simulink library "BrickPi"  (R2018b)
settings: Solver=VariableStepAuto  StartTime=0.0  StopTime=10.0  RelTol=1e-3
libraries: raspberrypilib x50, hdlsllib x27, xpcutilitieslib x18, $bdroot x1
(part 3 of 4)

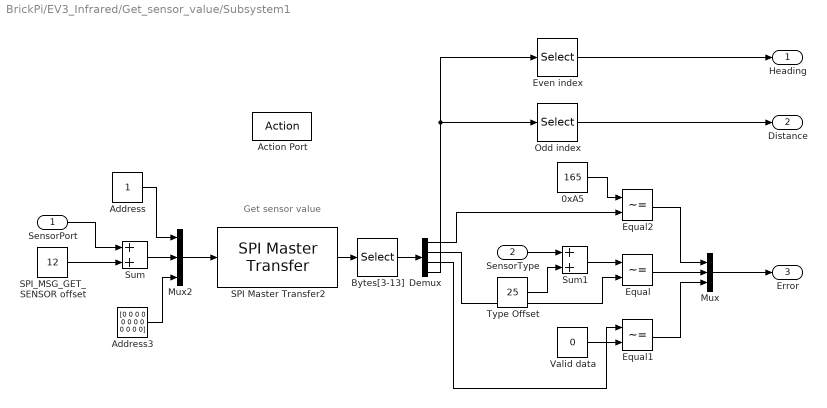
== system BrickPi/EV3_Infrared/Get_sensor_value/Subsystem1 ==
  note: Get sensor value
  SensorPort : Inport
  SensorType : Inport  Port=2  OutDataTypeStr=uint8
  Action Port : ActionPort  ActionType=case
  0xA5 : Constant  Value=165
  "Address " : Constant  OutDataTypeStr=uint8
  Address3 : Constant  Value=[0 0 0 0 0 0 0 0 0 0 0 0]  OutDataTypeStr=uint8
  Bytes[3-13] : Selector  IndexMode=Zero-based  InputPortWidth=14  IndexOptions=Index vector (dialog)  Indices=[3 4 5 6 7 8 9 10 11 12 13]  OutputSizes=1
  Demux : Demux
  Equal : RelationalOperator  Operator=~=  OutDataTypeStr=boolean  RndMeth=Simplest
  Equal1 : RelationalOperator  Operator=~=  OutDataTypeStr=boolean  RndMeth=Simplest
  Equal2 : RelationalOperator  Operator=~=  OutDataTypeStr=boolean  RndMeth=Simplest
  Even index : Selector  IndexMode=Zero-based  InputPortWidth=8  IndexOptions=Index vector (dialog)  Indices=[0 2 4 6]  OutputSizes=1
  Mux : Mux  Inputs=3
  Mux2 : Mux  Inputs=3
  Odd index : Selector  IndexMode=Zero-based  InputPortWidth=8  IndexOptions=Index vector (dialog)  Indices=[1 3 5 7]  OutputSizes=1
  SPI Master Transfer2 : raspberrypilib/SPI Master Transfer  Priority=6  BoardProperty=Pi 3 Model B  SPIModule=uint32(0)  Mode=Master  BusSpeed=1000000  Pin=SPI0_CE1  FirstBitToTransfer=Most significant bit (MSB)  ClockMode=0  BlockFunction=Transfer  RegisterAddress=0  OutputDataType=int8  OutputDataLength=1
      settings: SourceProductName=Simulink Support Package for Raspberry Pi Hardware  SourceProductBaseCode=RASPPI
  SPI_MSG_GET_ SENSOR offset : Constant  Value=12  OutMin=[1]  OutMax=[28]  OutDataTypeStr=uint8
  Sum : Sum  OutDataTypeStr=uint8
  Sum1 : Sum  OutDataTypeStr=uint8
  Type Offset : Constant  Value=25  OutDataTypeStr=uint8
  Valid data : Constant  Value=0  OutDataTypeStr=uint8
  Heading : Outport
  Distance : Outport  Port=2
  Error : Outport  Port=3
  wires:
  Equal2/1 -> Mux/1
  Demux/1 -> Equal2/2
  SPI_MSG_GET_ SENSOR offset/1 -> Sum/2
  Demux/3 -> Equal1/1
  Equal/1 -> Mux/2
  Demux/2 -> Equal/2
  Equal1/1 -> Mux/3
  "Address "/1 -> Mux2/1
  Valid data/1 -> Equal1/2
  Mux/1 -> Error/1
  Mux2/1 -> SPI Master Transfer2/1
  SPI Master Transfer2/1 -> Bytes[3-13]/1
  Bytes[3-13]/1 -> Demux/1
  Address3/1 -> Mux2/3
  SensorPort/1 -> Sum/1
  Sum/1 -> Mux2/2
  0xA5/1 -> Equal2/1
  Demux/4 -> Odd index/1, Even index/1
  Odd index/1 -> Distance/1
  Even index/1 -> Heading/1
  SensorType/1 -> Sum1/1
  Type Offset/1 -> Sum1/2
  Sum1/1 -> Equal/1

== system BrickPi/EV3_Infrared/Get_sensor_value/Subsystem2 ==
  note: Get sensor value
  SensorPort : Inport
  SensorType : Inport  Port=2  OutDataTypeStr=uint8
  Action Port : ActionPort  ActionType=case
  0xA5 : Constant  Value=165
  "Address " : Constant  OutDataTypeStr=uint8
  Address3 : Constant  Value=[0 0 0 0 0 0 0 0]  OutDataTypeStr=uint8
  Bytes[3-9] : Selector  IndexMode=Zero-based  InputPortWidth=10  IndexOptions=Index vector (dialog)  Indices=[3 4 5 6 7 8 9]  OutputSizes=1
  Demux : Demux
  Equal : RelationalOperator  Operator=~=  OutDataTypeStr=boolean  RndMeth=Simplest
  Equal1 : RelationalOperator  Operator=~=  OutDataTypeStr=boolean  RndMeth=Simplest
  Equal2 : RelationalOperator  Operator=~=  OutDataTypeStr=boolean  RndMeth=Simplest
  Mux : Mux  Inputs=3
  Mux2 : Mux  Inputs=3
  SPI Master Transfer2 : raspberrypilib/SPI Master Transfer  Priority=6  BoardProperty=Pi 3 Model B  SPIModule=uint32(0)  Mode=Master  BusSpeed=1000000  Pin=SPI0_CE1  FirstBitToTransfer=Most significant bit (MSB)  ClockMode=0  BlockFunction=Transfer  RegisterAddress=0  OutputDataType=int8  OutputDataLength=1
      settings: SourceProductName=Simulink Support Package for Raspberry Pi Hardware  SourceProductBaseCode=RASPPI
  SPI_MSG_GET_ SENSOR offset : Constant  Value=12  OutMin=[1]  OutMax=[28]  OutDataTypeStr=uint8
  Sum : Sum  OutDataTypeStr=uint8
  Sum1 : Sum  OutDataTypeStr=uint8
  Type Offset : Constant  Value=25  OutDataTypeStr=uint8
  Valid data : Constant  Value=0  OutDataTypeStr=uint8
  Remote : Outport
  Error : Outport  Port=2
  wires:
  Sum1/1 -> Equal/1
  Type Offset/1 -> Sum1/2
  SensorType/1 -> Sum1/1
  Demux/4 -> Remote/1
  0xA5/1 -> Equal2/1
  Sum/1 -> Mux2/2
  SensorPort/1 -> Sum/1
  Address3/1 -> Mux2/3
  Bytes[3-9]/1 -> Demux/1
  SPI Master Transfer2/1 -> Bytes[3-9]/1
  Mux2/1 -> SPI Master Transfer2/1
  Mux/1 -> Error/1
  Valid data/1 -> Equal1/2
  "Address "/1 -> Mux2/1
  Equal1/1 -> Mux/3
  Demux/2 -> Equal/2
  Equal/1 -> Mux/2
  Demux/3 -> Equal1/1
  SPI_MSG_GET_ SENSOR offset/1 -> Sum/2
  Demux/1 -> Equal2/2
  Equal2/1 -> Mux/1

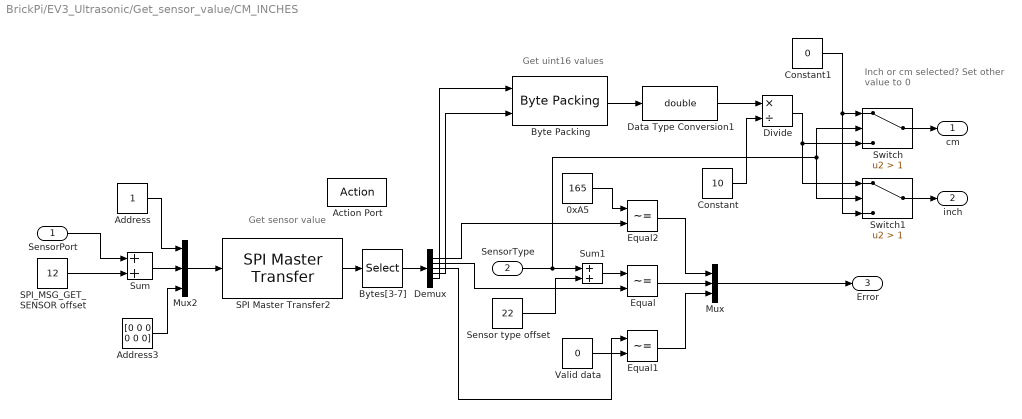
== system BrickPi/EV3_Ultrasonic/Get_sensor_value/CM_INCHES ==
  note: Inch or cm selected?
      | Set other value to 0
  note: Get uint16 values
  note: Get sensor value
  SensorPort : Inport
  SensorType : Inport  Port=2  OutDataTypeStr=uint8
  Action Port : ActionPort  ActionType=case
  0xA5 : Constant  Value=165
  "Address " : Constant  OutDataTypeStr=uint8
  Address3 : Constant  Value=[0 0 0 0 0 0]  OutDataTypeStr=uint8
  "Byte Packing " : xpcutilitieslib/Byte Packing   MaskPackedDataType=uint16  MaskUnpackedDataTypes={'uint8','uint8'}  MaskAlignment=1
  Bytes[3-7] : Selector  IndexMode=Zero-based  InputPortWidth=8  IndexOptions=Index vector (dialog)  Indices=[3 4 5 6 7]  OutputSizes=1
  Constant : Constant  Value=10
  Constant1 : Constant  Value=0
  Data Type Conversion1 : DataTypeConversion  OutDataTypeStr=double
  Demux : Demux  Outputs=5
  Divide : Product  Inputs=*/
  Equal : RelationalOperator  Operator=~=  OutDataTypeStr=boolean  RndMeth=Simplest
  Equal1 : RelationalOperator  Operator=~=  OutDataTypeStr=boolean  RndMeth=Simplest
  Equal2 : RelationalOperator  Operator=~=  OutDataTypeStr=boolean  RndMeth=Simplest
  Mux : Mux  Inputs=3
  Mux2 : Mux  Inputs=3
  SPI Master Transfer2 : raspberrypilib/SPI Master Transfer  Priority=6  BoardProperty=Pi 3 Model B  SPIModule=uint32(0)  Mode=Master  BusSpeed=1000000  Pin=SPI0_CE1  FirstBitToTransfer=Most significant bit (MSB)  ClockMode=0  BlockFunction=Transfer  RegisterAddress=0  OutputDataType=int8  OutputDataLength=1
      settings: SourceProductName=Simulink Support Package for Raspberry Pi Hardware  SourceProductBaseCode=RASPPI
  SPI_MSG_GET_ SENSOR offset : Constant  Value=12  OutMin=[1]  OutMax=[28]  OutDataTypeStr=uint8
  Sensor type offset : Constant  Value=22  OutDataTypeStr=uint8
  Sum : Sum  OutDataTypeStr=uint8
  Sum1 : Sum
  Switch : Switch  Criteria=u2 > Threshold  Threshold=1
  Switch1 : Switch  Criteria=u2 > Threshold  Threshold=1
  Valid data : Constant  Value=0  OutDataTypeStr=uint8
  cm : Outport
  inch : Outport  Port=2
  Error : Outport  Port=3
  wires:
  0xA5/1 -> Equal2/1
  Equal1/1 -> Mux/3
  Equal2/1 -> Mux/1
  SPI Master Transfer2/1 -> Bytes[3-7]/1
  SensorType/1 -> Switch/2, Switch1/2, Sum1/1
  "Address "/1 -> Mux2/1
  Sum/1 -> Mux2/2
  Sensor type offset/1 -> Sum1/2
  Address3/1 -> Mux2/3
  Demux/2 -> Equal/2
  Mux2/1 -> SPI Master Transfer2/1
  Valid data/1 -> Equal1/2
  Demux/3 -> Equal1/1
  Sum1/1 -> Equal/1
  Mux/1 -> Error/1
  SPI_MSG_GET_ SENSOR offset/1 -> Sum/2
  Demux/1 -> Equal2/2
  Bytes[3-7]/1 -> Demux/1
  SensorPort/1 -> Sum/1
  Equal/1 -> Mux/2
  "Byte Packing "/1 -> Data Type Conversion1/1
  Data Type Conversion1/1 -> Divide/1
  Constant/1 -> Divide/2
  Switch/1 -> cm/1
  Switch1/1 -> inch/1
  Divide/1 -> Switch/3, Switch1/1
  Constant1/1 -> Switch/1, Switch1/3
  Demux/4 -> "Byte Packing "/2
  Demux/5 -> "Byte Packing "/1

== system BrickPi/EV3_Ultrasonic/Get_sensor_value/LISTEN ==
  note: Get sensor value
  SensorPort : Inport
  Action Port : ActionPort  ActionType=case
  0xA5 : Constant  Value=165
  "Address " : Constant  OutDataTypeStr=uint8
  Address3 : Constant  Value=[0 0 0 0 0]  OutDataTypeStr=uint8
  Bytes[3-6] : Selector  IndexMode=Zero-based  InputPortWidth=7  IndexOptions=Index vector (dialog)  Indices=[3 4 5 6]  OutputSizes=1
  Cast To Boolean : DataTypeConversion  OutDataTypeStr=boolean
  Demux : Demux
  Mux : Mux  Inputs=3
  Mux2 : Mux  Inputs=3
  NAND : Logic  Operator=NAND  IconShape=distinctive  AllPortsSameDT=off  OutDataTypeStr=boolean
  NAND1 : Logic  Operator=NAND  IconShape=distinctive  AllPortsSameDT=off  OutDataTypeStr=boolean
  OR1 : Logic  Operator=OR  IconShape=distinctive  AllPortsSameDT=off  OutDataTypeStr=boolean
  SPI Master Transfer2 : raspberrypilib/SPI Master Transfer  Priority=6  BoardProperty=Pi 3 Model B  SPIModule=uint32(0)  Mode=Master  BusSpeed=1000000  Pin=SPI0_CE1  FirstBitToTransfer=Most significant bit (MSB)  ClockMode=0  BlockFunction=Transfer  RegisterAddress=0  OutputDataType=int8  OutputDataLength=1
      settings: SourceProductName=Simulink Support Package for Raspberry Pi Hardware  SourceProductBaseCode=RASPPI
  SPI_MSG_GET_ SENSOR offset : Constant  Value=12  OutMin=[1]  OutMax=[28]  OutDataTypeStr=uint8
  Sum : Sum  OutDataTypeStr=uint8
  ULTRASONIC_LISTEN : Constant  Value=25  OutMin=[1]  OutMax=[28]  OutDataTypeStr=uint8
  Valid data : Constant  Value=0  OutDataTypeStr=uint8
  presence : Outport
  Error : Outport  Port=2
  wires:
  ULTRASONIC_LISTEN/1 -> NAND1/1
  NAND/1 -> Mux/1
  SPI Master Transfer2/1 -> Bytes[3-6]/1
  Valid data/1 -> OR1/2
  Sum/1 -> Mux2/2
  0xA5/1 -> NAND/1
  Demux/3 -> OR1/1
  Mux2/1 -> SPI Master Transfer2/1
  Address3/1 -> Mux2/3
  NAND1/1 -> Mux/2
  Demux/2 -> NAND1/2
  "Address "/1 -> Mux2/1
  Demux/4 -> Cast To Boolean/1
  Demux/1 -> NAND/2
  SensorPort/1 -> Sum/1
  SPI_MSG_GET_ SENSOR offset/1 -> Sum/2
  Mux/1 -> Error/1
  OR1/1 -> Mux/3
  Bytes[3-6]/1 -> Demux/1
  Cast To Boolean/1 -> presence/1

== system BrickPi/Motor_Encoder/Get Encoder Value/Switch Case Action Subsystem ==
  note: Change from zero to nonzero?
  note: Change in input signal?
  ExtSignal : Inport
  MotorPort : Inport  Port=2
  Action Port : ActionPort  ActionType=case
  AND : Logic  IconShape=distinctive  AllPortsSameDT=off  OutDataTypeStr=boolean
  Constant : Constant  Value=0
  Equal : RelationalOperator  Operator=~=  OutDataTypeStr=boolean  RndMeth=Simplest
  Equal1 : RelationalOperator  Operator=~=  OutDataTypeStr=boolean  RndMeth=Simplest
  Memory : Memory
  Subsystem : Subsystem
  wires:
  Equal/1 -> AND/1
  Equal1/1 -> AND/2
  Memory/1 -> Equal/1
  Constant/1 -> Equal1/2
  ExtSignal/1 -> Equal1/1, Equal/2, Memory/1
  AND/1 -> Subsystem/Enable
  MotorPort/1 -> Subsystem/1(MotorPort)

== system BrickPi/Motor_Encoder/Reset Encoder once/Encoder ==
  note: Get motor encoder
  MotorPort : Inport
  0xA5 : Constant  Value=165
  "Address " : Constant  OutDataTypeStr=uint8
  Address3 : Constant  Value=[0 0 0 0 0 0 0 0]  OutDataTypeStr=uint8
  "Byte Packing " : xpcutilitieslib/Byte Packing   MaskPackedDataType=int32  MaskUnpackedDataTypes={'uint8', 'uint8', 'uint8', 'uint8'}  MaskAlignment=1
  Bytes[3-7] : Selector  IndexMode=Zero-based  InputPortWidth=10  IndexOptions=Index vector (dialog)  Indices=[3 4 5 6 7]  OutputSizes=1
  Demux : Demux  Outputs=5
  Mux2 : Mux  Inputs=3
  NAND : Logic  Operator=NAND  IconShape=distinctive  AllPortsSameDT=off  OutDataTypeStr=boolean
  SPI Master Transfer2 : raspberrypilib/SPI Master Transfer  Priority=6  BoardProperty=Pi 3 Model B  SPIModule=uint32(0)  Mode=Master  BusSpeed=1000000  Pin=SPI0_CE1  FirstBitToTransfer=Most significant bit (MSB)  ClockMode=0  BlockFunction=Transfer  RegisterAddress=0  OutputDataType=int8  OutputDataLength=1
      settings: SourceProductName=Simulink Support Package for Raspberry Pi Hardware  SourceProductBaseCode=RASPPI
  SPI_MSG_GET_ MOTOR_ENCODER offset : Constant  Value=29  OutDataTypeStr=uint8
  Sum : Sum  OutDataTypeStr=uint8
  Value : Outport
  Error : Outport  Port=2
  wires:
  Address3/1 -> Mux2/3
  NAND/1 -> Error/1
  Sum/1 -> Mux2/2
  Mux2/1 -> SPI Master Transfer2/1
  MotorPort/1 -> Sum/1
  Demux/5 -> "Byte Packing "/1
  "Address "/1 -> Mux2/1
  Demux/4 -> "Byte Packing "/2
  Demux/3 -> "Byte Packing "/3
  Demux/1 -> NAND/2
  0xA5/1 -> NAND/1
  Demux/2 -> "Byte Packing "/4
  "Byte Packing "/1 -> Value/1
  Bytes[3-7]/1 -> Demux/1
  SPI Master Transfer2/1 -> Bytes[3-7]/1
  SPI_MSG_GET_ MOTOR_ENCODER offset/1 -> Sum/2

== system BrickPi/Motor_Encoder/Reset Encoder once/Motor_Offset ==
  note: Set offset value
  Offset : Inport  OutDataTypeStr=int32
  MotorPort : Inport  Port=2  OutDataTypeStr=uint8
  "Address " : Constant  OutDataTypeStr=uint8
  Bit Shift : hdlsllib/Logic and Bit Operations/Bit Shift  mode=Shift Right Logical  N=24
      settings: SourceProductName=HDL Coder  SourceProductBaseCode=HD
  Bit Shift1 : hdlsllib/Logic and Bit Operations/Bit Shift  mode=Shift Right Logical  N=16
      settings: SourceProductName=HDL Coder  SourceProductBaseCode=HD
  Bit Shift2 : hdlsllib/Logic and Bit Operations/Bit Shift  mode=Shift Right Logical  N=8
      settings: SourceProductName=HDL Coder  SourceProductBaseCode=HD
  Constant2 : Constant  OutDataTypeStr=uint8
  Constant3 : Constant  OutDataTypeStr=uint8
  Data Type Conversion{,1..3} (4 alike) : DataTypeConversion  OutDataTypeStr=uint8
  Mux2 : Mux  Inputs=7
  SPI Master Transfer2 : raspberrypilib/SPI Master Transfer  Priority=6  BoardProperty=Pi 3 Model B  SPIModule=uint32(0)  Mode=Master  BusSpeed=1000000  Pin=SPI0_CE1  FirstBitToTransfer=Most significant bit (MSB)  ClockMode=0  BlockFunction=Transfer  RegisterAddress=0  OutputDataType=int8  OutputDataLength=1
      settings: SourceProductName=Simulink Support Package for Raspberry Pi Hardware  SourceProductBaseCode=RASPPI
  SPI_MSG_ OFFSET_ENCODER : Constant  Value=29  OutMin=[1]  OutDataTypeStr=uint8
  Shift Arithmetic : ArithShift  BitShiftNumberSource=Input port  BitShiftNumber=8  BitShiftDirection=Left
      settings: InputPortMap=u0,p1
  Subtract : Sum  Inputs=+-
  Terminator : Terminator
  wires:
  Data Type Conversion/1 -> Mux2/4
  Data Type Conversion2/1 -> Mux2/6
  Offset/1 -> Bit Shift1/1, Bit Shift2/1, Data Type Conversion3/1, Bit Shift/1
  Constant2/1 -> Shift Arithmetic/1
  Bit Shift2/1 -> Data Type Conversion2/1
  Constant3/1 -> Subtract/2
  Bit Shift/1 -> Data Type Conversion/1
  Mux2/1 -> SPI Master Transfer2/1
  SPI Master Transfer2/1 -> Terminator/1
  Data Type Conversion3/1 -> Mux2/7
  Subtract/1 -> Shift Arithmetic/2
  MotorPort/1 -> Subtract/1
  Bit Shift1/1 -> Data Type Conversion1/1
  Data Type Conversion1/1 -> Mux2/5
  SPI_MSG_ OFFSET_ENCODER/1 -> Mux2/2
  "Address "/1 -> Mux2/1
  Shift Arithmetic/1 -> Mux2/3

== system BrickPi/Motor_Power/Subsystem/Set_DPS ==
  note: Get sensor value
  DPS : Inport  OutDataTypeStr=int16
  Action Port : ActionPort  ActionType=case
  "Address " : Constant  OutDataTypeStr=uint8
  Bit Shift : hdlsllib/Logic and Bit Operations/Bit Shift  mode=Shift Right Logical  N=8
      settings: SourceProductName=HDL Coder  SourceProductBaseCode=HD
  Constant2 : Constant  OutDataTypeStr=uint8
  Constant3 : Constant  OutDataTypeStr=uint8
  Data Type Conversion : DataTypeConversion  OutDataTypeStr=uint8
  Data Type Conversion1 : DataTypeConversion  OutDataTypeStr=uint8
  MotorPort : Constant  Value=MotorPort  OutDataTypeStr=uint8
  Mux2 : Mux  Inputs=5
  SPI Master Transfer2 : raspberrypilib/SPI Master Transfer  Priority=6  BoardProperty=Pi 3 Model B  SPIModule=uint32(0)  Mode=Master  BusSpeed=1000000  Pin=SPI0_CE1  FirstBitToTransfer=Most significant bit (MSB)  ClockMode=0  BlockFunction=Transfer  RegisterAddress=0  OutputDataType=int8  OutputDataLength=1
      settings: SourceProductName=Simulink Support Package for Raspberry Pi Hardware  SourceProductBaseCode=RASPPI
  SPI_MSG_SET_ MOTOR_DPS : Constant  Value=25  OutMin=[1]  OutMax=[28]  OutDataTypeStr=uint8
  Shift Arithmetic : ArithShift  BitShiftNumberSource=Input port  BitShiftNumber=8  BitShiftDirection=Left
      settings: InputPortMap=u0,p1
  Subtract : Sum  Inputs=+-
  Terminator : Terminator
  wires:
  Subtract/1 -> Shift Arithmetic/2
  Shift Arithmetic/1 -> Mux2/3
  Mux2/1 -> SPI Master Transfer2/1
  Constant3/1 -> Subtract/2
  SPI_MSG_SET_ MOTOR_DPS/1 -> Mux2/2
  SPI Master Transfer2/1 -> Terminator/1
  MotorPort/1 -> Subtract/1
  Constant2/1 -> Shift Arithmetic/1
  "Address "/1 -> Mux2/1
  Bit Shift/1 -> Data Type Conversion/1
  Data Type Conversion1/1 -> Mux2/5
  Data Type Conversion/1 -> Mux2/4
  DPS/1 -> Data Type Conversion1/1, Bit Shift/1

== system BrickPi/Motor_Power/Subsystem/Set_Limit ==
  note: Get sensor value
  Power : Inport  OutDataTypeStr=int8
  DPS : Inport  Port=2  OutDataTypeStr=int16
  Action Port : ActionPort  ActionType=case
  "Address " : Constant  OutDataTypeStr=uint8
  Bit Shift : hdlsllib/Logic and Bit Operations/Bit Shift  mode=Shift Right Logical  N=8
      settings: SourceProductName=HDL Coder  SourceProductBaseCode=HD
  Constant2 : Constant  OutDataTypeStr=uint8
  Constant3 : Constant  OutDataTypeStr=uint8
  Data Type Conversion : DataTypeConversion  OutDataTypeStr=uint8
  Data Type Conversion1 : DataTypeConversion  OutDataTypeStr=uint8
  Data Type Conversion2 : DataTypeConversion  OutDataTypeStr=uint8
  MotorPort : Constant  Value=MotorPort  OutDataTypeStr=uint8
  Mux2 : Mux  Inputs=6
  SPI Master Transfer2 : raspberrypilib/SPI Master Transfer  Priority=6  BoardProperty=Pi 3 Model B  SPIModule=uint32(0)  Mode=Master  BusSpeed=1000000  Pin=SPI0_CE1  FirstBitToTransfer=Most significant bit (MSB)  ClockMode=0  BlockFunction=Transfer  RegisterAddress=0  OutputDataType=int8  OutputDataLength=1
      settings: SourceProductName=Simulink Support Package for Raspberry Pi Hardware  SourceProductBaseCode=RASPPI
  SPI_MSG_SET_ MOTOR_LIMITS : Constant  Value=28  OutMin=[1]  OutMax=[28]  OutDataTypeStr=uint8
  Shift Arithmetic : ArithShift  BitShiftNumberSource=Input port  BitShiftNumber=8  BitShiftDirection=Left
      settings: InputPortMap=u0,p1
  Subtract : Sum  Inputs=+-
  Terminator : Terminator
  wires:
  Subtract/1 -> Shift Arithmetic/2
  Shift Arithmetic/1 -> Mux2/3
  Mux2/1 -> SPI Master Transfer2/1
  Constant3/1 -> Subtract/2
  SPI_MSG_SET_ MOTOR_LIMITS/1 -> Mux2/2
  SPI Master Transfer2/1 -> Terminator/1
  MotorPort/1 -> Subtract/1
  Constant2/1 -> Shift Arithmetic/1
  "Address "/1 -> Mux2/1
  Bit Shift/1 -> Data Type Conversion/1
  Data Type Conversion1/1 -> Mux2/6
  Data Type Conversion/1 -> Mux2/5
  DPS/1 -> Data Type Conversion1/1, Bit Shift/1
  Power/1 -> Data Type Conversion2/1
  Data Type Conversion2/1 -> Mux2/4

== system BrickPi/Motor_Power/Subsystem/Set_Position ==
  note: Get sensor value
  Position : Inport  OutDataTypeStr=int32
  Action Port : ActionPort  ActionType=case
  "Address " : Constant  OutDataTypeStr=uint8
  Bit Shift : hdlsllib/Logic and Bit Operations/Bit Shift  mode=Shift Right Logical  N=24
      settings: SourceProductName=HDL Coder  SourceProductBaseCode=HD
  Bit Shift1 : hdlsllib/Logic and Bit Operations/Bit Shift  mode=Shift Right Logical  N=16
      settings: SourceProductName=HDL Coder  SourceProductBaseCode=HD
  Bit Shift2 : hdlsllib/Logic and Bit Operations/Bit Shift  mode=Shift Right Logical  N=8
      settings: SourceProductName=HDL Coder  SourceProductBaseCode=HD
  Constant2 : Constant  OutDataTypeStr=uint8
  Constant3 : Constant  OutDataTypeStr=uint8
  Data Type Conversion{,1..3} (4 alike) : DataTypeConversion  OutDataTypeStr=uint8
  MotorPort : Constant  Value=MotorPort  OutDataTypeStr=uint8
  Mux2 : Mux  Inputs=7
  SPI Master Transfer2 : raspberrypilib/SPI Master Transfer  Priority=6  BoardProperty=Pi 3 Model B  SPIModule=uint32(0)  Mode=Master  BusSpeed=1000000  Pin=SPI0_CE1  FirstBitToTransfer=Most significant bit (MSB)  ClockMode=0  BlockFunction=Transfer  RegisterAddress=0  OutputDataType=int8  OutputDataLength=1
      settings: SourceProductName=Simulink Support Package for Raspberry Pi Hardware  SourceProductBaseCode=RASPPI
  SPI_MSG_SET_ MOTOR_POSITION : Constant  Value=22  OutMin=[1]  OutMax=[28]  OutDataTypeStr=uint8
  Shift Arithmetic : ArithShift  BitShiftNumberSource=Input port  BitShiftNumber=8  BitShiftDirection=Left
      settings: InputPortMap=u0,p1
  Subtract : Sum  Inputs=+-
  Terminator : Terminator
  wires:
  Subtract/1 -> Shift Arithmetic/2
  Position/1 -> Data Type Conversion3/1, Bit Shift2/1, Bit Shift1/1, Bit Shift/1
  Shift Arithmetic/1 -> Mux2/3
  Mux2/1 -> SPI Master Transfer2/1
  Constant3/1 -> Subtract/2
  SPI_MSG_SET_ MOTOR_POSITION/1 -> Mux2/2
  SPI Master Transfer2/1 -> Terminator/1
  MotorPort/1 -> Subtract/1
  Constant2/1 -> Shift Arithmetic/1
  Bit Shift2/1 -> Data Type Conversion2/1
  "Address "/1 -> Mux2/1
  Data Type Conversion3/1 -> Mux2/7
  Bit Shift/1 -> Data Type Conversion/1
  Data Type Conversion1/1 -> Mux2/5
  Data Type Conversion/1 -> Mux2/4
  Bit Shift1/1 -> Data Type Conversion1/1
  Data Type Conversion2/1 -> Mux2/6

== system BrickPi/Motor_Power/Subsystem/Set_Power ==
  note: Get sensor value
  Power : Inport  OutDataTypeStr=int8
  Action Port : ActionPort  ActionType=case
  "Address " : Constant  OutDataTypeStr=uint8
  Constant2 : Constant  OutDataTypeStr=uint8
  Constant3 : Constant  OutDataTypeStr=uint8
  Data Type Conversion : DataTypeConversion  OutDataTypeStr=uint8
  MotorPort : Constant  Value=MotorPort  OutDataTypeStr=uint8
  Mux2 : Mux
  SPI Master Transfer2 : raspberrypilib/SPI Master Transfer  Priority=6  BoardProperty=Pi 3 Model B  SPIModule=uint32(0)  Mode=Master  BusSpeed=1000000  Pin=SPI0_CE1  FirstBitToTransfer=Most significant bit (MSB)  ClockMode=0  BlockFunction=Transfer  RegisterAddress=0  OutputDataType=int8  OutputDataLength=1
      settings: SourceProductName=Simulink Support Package for Raspberry Pi Hardware  SourceProductBaseCode=RASPPI
  SPI_MSG_SET_ MOTOR_POWER : Constant  Value=21  OutMin=[1]  OutMax=[28]  OutDataTypeStr=uint8
  Shift Arithmetic : ArithShift  BitShiftNumberSource=Input port  BitShiftNumber=8  BitShiftDirection=Left
      settings: InputPortMap=u0,p1
  Subtract : Sum  Inputs=+-
  Terminator : Terminator
  wires:
  Subtract/1 -> Shift Arithmetic/2
  Mux2/1 -> SPI Master Transfer2/1
  "Address "/1 -> Mux2/1
  Constant3/1 -> Subtract/2
  MotorPort/1 -> Subtract/1
  Constant2/1 -> Shift Arithmetic/1
  SPI_MSG_SET_ MOTOR_POWER/1 -> Mux2/2
  Data Type Conversion/1 -> Mux2/4
  SPI Master Transfer2/1 -> Terminator/1
  Shift Arithmetic/1 -> Mux2/3
  Power/1 -> Data Type Conversion/1

== system BrickPi/Motor_Status/Get motor values/Switch Case Action Subsystem ==
  note: Change from zero to nonzero?
  note: Change in input signal?
  ExtSignal : Inport
  MotorPort : Inport  Port=2
  Action Port : ActionPort  ActionType=case
  AND : Logic  IconShape=distinctive  AllPortsSameDT=off  OutDataTypeStr=boolean
  Constant : Constant  Value=0
  Equal : RelationalOperator  Operator=~=  OutDataTypeStr=boolean  RndMeth=Simplest
  Equal1 : RelationalOperator  Operator=~=  OutDataTypeStr=boolean  RndMeth=Simplest
  Memory : Memory
  Subsystem : Subsystem
  wires:
  Equal/1 -> AND/1
  Equal1/1 -> AND/2
  Memory/1 -> Equal/1
  Constant/1 -> Equal1/2
  ExtSignal/1 -> Equal1/1, Equal/2, Memory/1
  AND/1 -> Subsystem/Enable
  MotorPort/1 -> Subsystem/1(MotorPort)

== system BrickPi/Motor_Status/Reset Encoder once/Encoder ==
  note: Get motor encoder
  MotorPort : Inport
  0xA5 : Constant  Value=165
  "Address " : Constant  OutDataTypeStr=uint8
  Address3 : Constant  Value=[0 0 0 0 0 0 0 0]  OutDataTypeStr=uint8
  "Byte Packing " : xpcutilitieslib/Byte Packing   MaskPackedDataType=int32  MaskUnpackedDataTypes={'uint8', 'uint8', 'uint8', 'uint8'}  MaskAlignment=1
  Bytes[3-7] : Selector  IndexMode=Zero-based  InputPortWidth=10  IndexOptions=Index vector (dialog)  Indices=[3 4 5 6 7]  OutputSizes=1
  Demux : Demux  Outputs=5
  Mux2 : Mux  Inputs=3
  NAND : Logic  Operator=NAND  IconShape=distinctive  AllPortsSameDT=off  OutDataTypeStr=boolean
  SPI Master Transfer2 : raspberrypilib/SPI Master Transfer  Priority=6  BoardProperty=Pi 3 Model B  SPIModule=uint32(0)  Mode=Master  BusSpeed=1000000  Pin=SPI0_CE1  FirstBitToTransfer=Most significant bit (MSB)  ClockMode=0  BlockFunction=Transfer  RegisterAddress=0  OutputDataType=int8  OutputDataLength=1
      settings: SourceProductName=Simulink Support Package for Raspberry Pi Hardware  SourceProductBaseCode=RASPPI
  SPI_MSG_GET_ MOTOR_ENCODER offset : Constant  Value=29  OutDataTypeStr=uint8
  Sum : Sum  OutDataTypeStr=uint8
  Value : Outport
  Error : Outport  Port=2
  wires:
  Address3/1 -> Mux2/3
  NAND/1 -> Error/1
  Sum/1 -> Mux2/2
  Mux2/1 -> SPI Master Transfer2/1
  MotorPort/1 -> Sum/1
  Demux/5 -> "Byte Packing "/1
  "Address "/1 -> Mux2/1
  Demux/4 -> "Byte Packing "/2
  Demux/3 -> "Byte Packing "/3
  Demux/1 -> NAND/2
  0xA5/1 -> NAND/1
  Demux/2 -> "Byte Packing "/4
  "Byte Packing "/1 -> Value/1
  Bytes[3-7]/1 -> Demux/1
  SPI Master Transfer2/1 -> Bytes[3-7]/1
  SPI_MSG_GET_ MOTOR_ENCODER offset/1 -> Sum/2

== system BrickPi/Motor_Status/Reset Encoder once/Motor_Offset ==
  note: Set offset value
  Offset : Inport  OutDataTypeStr=int32
  MotorPort : Inport  Port=2  OutDataTypeStr=uint8
  "Address " : Constant  OutDataTypeStr=uint8
  Bit Shift : hdlsllib/Logic and Bit Operations/Bit Shift  mode=Shift Right Logical  N=24
      settings: SourceProductName=HDL Coder  SourceProductBaseCode=HD
  Bit Shift1 : hdlsllib/Logic and Bit Operations/Bit Shift  mode=Shift Right Logical  N=16
      settings: SourceProductName=HDL Coder  SourceProductBaseCode=HD
  Bit Shift2 : hdlsllib/Logic and Bit Operations/Bit Shift  mode=Shift Right Logical  N=8
      settings: SourceProductName=HDL Coder  SourceProductBaseCode=HD
  Constant2 : Constant  OutDataTypeStr=uint8
  Constant3 : Constant  OutDataTypeStr=uint8
  Data Type Conversion{,1..3} (4 alike) : DataTypeConversion  OutDataTypeStr=uint8
  Mux2 : Mux  Inputs=7
  SPI Master Transfer2 : raspberrypilib/SPI Master Transfer  Priority=6  BoardProperty=Pi 3 Model B  SPIModule=uint32(0)  Mode=Master  BusSpeed=1000000  Pin=SPI0_CE1  FirstBitToTransfer=Most significant bit (MSB)  ClockMode=0  BlockFunction=Transfer  RegisterAddress=0  OutputDataType=int8  OutputDataLength=1
      settings: SourceProductName=Simulink Support Package for Raspberry Pi Hardware  SourceProductBaseCode=RASPPI
  SPI_MSG_ OFFSET_ENCODER : Constant  Value=29  OutMin=[1]  OutDataTypeStr=uint8
  Shift Arithmetic : ArithShift  BitShiftNumberSource=Input port  BitShiftNumber=8  BitShiftDirection=Left
      settings: InputPortMap=u0,p1
  Subtract : Sum  Inputs=+-
  Terminator : Terminator
  wires:
  Data Type Conversion/1 -> Mux2/4
  Data Type Conversion2/1 -> Mux2/6
  Offset/1 -> Bit Shift1/1, Bit Shift2/1, Data Type Conversion3/1, Bit Shift/1
  Constant2/1 -> Shift Arithmetic/1
  Bit Shift2/1 -> Data Type Conversion2/1
  Constant3/1 -> Subtract/2
  Bit Shift/1 -> Data Type Conversion/1
  Mux2/1 -> SPI Master Transfer2/1
  SPI Master Transfer2/1 -> Terminator/1
  Data Type Conversion3/1 -> Mux2/7
  Subtract/1 -> Shift Arithmetic/2
  MotorPort/1 -> Subtract/1
  Bit Shift1/1 -> Data Type Conversion1/1
  Data Type Conversion1/1 -> Mux2/5
  SPI_MSG_ OFFSET_ENCODER/1 -> Mux2/2
  "Address "/1 -> Mux2/1
  Shift Arithmetic/1 -> Mux2/3

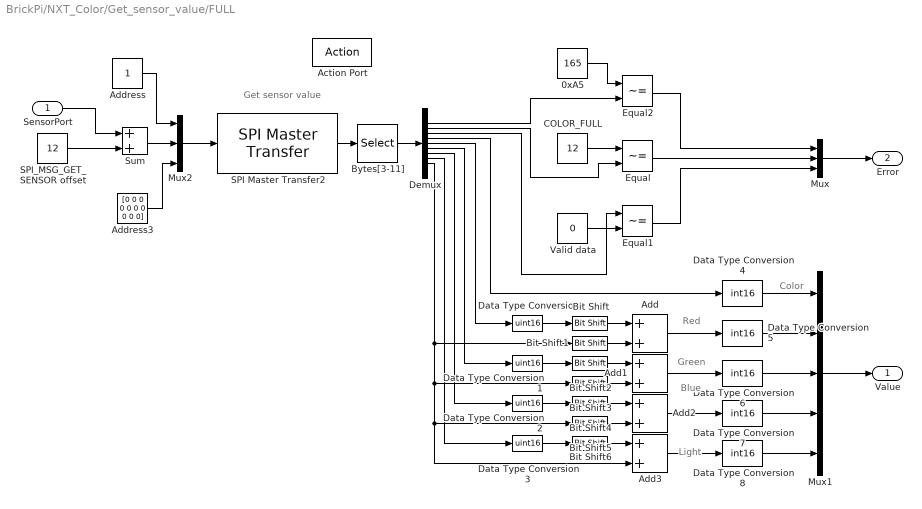
== system BrickPi/NXT_Color/Get_sensor_value/FULL ==
  note: Color
  note: Get sensor value
  note: Red
  note: Green
  note: Blue
  note: Light
  SensorPort : Inport
  Action Port : ActionPort  ActionType=case
  0xA5 : Constant  Value=165
  Add{,1..3} (4 alike) : Sum  OutDataTypeStr=uint16
  "Address " : Constant  OutDataTypeStr=uint8
  Address3 : Constant  Value=[0 0 0 0 0 0 0 0 0 0]  OutDataTypeStr=uint8
  Bit Shift{,2,4,6} (4 alike) : hdlsllib/Logic and Bit Operations/Bit Shift  mode=Shift Left Logical  N=2
      settings: SourceProductName=HDL Coder  SourceProductBaseCode=HD
  Bit Shift1 : hdlsllib/Logic and Bit Operations/Bit Shift  mode=Shift Right Logical  N=6
      settings: SourceProductName=HDL Coder  SourceProductBaseCode=HD
  Bit Shift3 : hdlsllib/Logic and Bit Operations/Bit Shift  mode=Shift Right Logical  N=4
      settings: SourceProductName=HDL Coder  SourceProductBaseCode=HD
  Bit Shift5 : hdlsllib/Logic and Bit Operations/Bit Shift  mode=Shift Right Logical  N=2
      settings: SourceProductName=HDL Coder  SourceProductBaseCode=HD
  Bytes[3-11] : Selector  IndexMode=Zero-based  InputPortWidth=12  IndexOptions=Index vector (dialog)  Indices=[3 4 5 6 7 8 9 10 11]  OutputSizes=1
  COLOR_FULL : Constant  Value=12  OutDataTypeStr=uint8
  Data Type Conversion{,1..3} (4 alike) : DataTypeConversion  OutDataTypeStr=uint16
  Data Type Conversion{4..8} (5 alike) : DataTypeConversion  OutDataTypeStr=int16
  Demux : Demux  Outputs=9
  Equal : RelationalOperator  Operator=~=  OutDataTypeStr=boolean  RndMeth=Simplest
  Equal1 : RelationalOperator  Operator=~=  OutDataTypeStr=boolean  RndMeth=Simplest
  Equal2 : RelationalOperator  Operator=~=  OutDataTypeStr=boolean  RndMeth=Simplest
  Mux : Mux  Inputs=3
  Mux1 : Mux  Inputs=5
  Mux2 : Mux  Inputs=3
  SPI Master Transfer2 : raspberrypilib/SPI Master Transfer  Priority=6  BoardProperty=Pi 3 Model B  SPIModule=uint32(0)  Mode=Master  BusSpeed=1000000  Pin=SPI0_CE1  FirstBitToTransfer=Most significant bit (MSB)  ClockMode=0  BlockFunction=Transfer  RegisterAddress=0  OutputDataType=int8  OutputDataLength=1
      settings: SourceProductName=Simulink Support Package for Raspberry Pi Hardware  SourceProductBaseCode=RASPPI
  SPI_MSG_GET_ SENSOR offset : Constant  Value=12  OutMin=[1]  OutMax=[28]  OutDataTypeStr=uint8
  Sum : Sum  OutDataTypeStr=uint8
  Valid data : Constant  Value=0  OutDataTypeStr=uint8
  Value : Outport
  Error : Outport  Port=2
  wires:
  SensorPort/1 -> Sum/1
  0xA5/1 -> Equal2/1
  Equal2/1 -> Mux/1
  Mux/1 -> Error/1
  Equal/1 -> Mux/2
  Address3/1 -> Mux2/3
  Demux/3 -> Equal1/1
  Valid data/1 -> Equal1/2
  Demux/2 -> Equal/2
  Bit Shift/1 -> Add/1
  Demux/1 -> Equal2/2
  Data Type Conversion/1 -> Bit Shift/1
  Sum/1 -> Mux2/2
  SPI_MSG_GET_ SENSOR offset/1 -> Sum/2
  Mux2/1 -> SPI Master Transfer2/1
  Equal1/1 -> Mux/3
  SPI Master Transfer2/1 -> Bytes[3-11]/1
  "Address "/1 -> Mux2/1
  Bytes[3-11]/1 -> Demux/1
  COLOR_FULL/1 -> Equal/1
  Demux/4 -> Data Type Conversion4/1
  Mux1/1 -> Value/1
  Bit Shift1/1 -> Add/2
  Demux/5 -> Data Type Conversion/1
  Add/1 -> Data Type Conversion5/1
  Bit Shift3/1 -> Add1/2
  Bit Shift2/1 -> Add1/1
  Data Type Conversion1/1 -> Bit Shift2/1
  Add1/1 -> Data Type Conversion6/1
  Demux/6 -> Data Type Conversion1/1
  Bit Shift5/1 -> Add2/2
  Data Type Conversion2/1 -> Bit Shift4/1
  Bit Shift4/1 -> Add2/1
  Demux/7 -> Data Type Conversion2/1
  Demux/9 -> Add3/2, Bit Shift5/1, Bit Shift3/1, Bit Shift1/1
  Data Type Conversion3/1 -> Bit Shift6/1
  Bit Shift6/1 -> Add3/1
  Demux/8 -> Data Type Conversion3/1
  Add2/1 -> Data Type Conversion7/1
  Add3/1 -> Data Type Conversion8/1
  Data Type Conversion4/1 -> Mux1/1
  Data Type Conversion5/1 -> Mux1/2
  Data Type Conversion6/1 -> Mux1/3
  Data Type Conversion7/1 -> Mux1/4
  Data Type Conversion8/1 -> Mux1/5

== system BrickPi/NXT_Color/Get_sensor_value/R_G_B_OFF ==
  note: Get sensor value
  SensorPort : Inport
  SensorType : Inport  Port=2  OutDataTypeStr=uint8
  Action Port : ActionPort  ActionType=case
  0xA5 : Constant  Value=165
  "Address " : Constant  OutDataTypeStr=uint8
  Address3 : Constant  Value=[0 0 0 0 0 0]  OutDataTypeStr=uint8
  "Byte Packing " : xpcutilitieslib/Byte Packing   MaskPackedDataType=int16  MaskUnpackedDataTypes={'uint8', 'uint8'}  MaskAlignment=1
  Bytes[3-6] : Selector  IndexMode=Zero-based  InputPortWidth=8  IndexOptions=Index vector (dialog)  Indices=[3 4 5 6 7]  OutputSizes=1
  Constant : Constant  Value=0  OutDataTypeStr=int16
  Demux : Demux  Outputs=5
  Equal : RelationalOperator  Operator=~=  OutDataTypeStr=boolean  RndMeth=Simplest
  Equal1 : RelationalOperator  Operator=~=  OutDataTypeStr=boolean  RndMeth=Simplest
  Equal2 : RelationalOperator  Operator=~=  OutDataTypeStr=boolean  RndMeth=Simplest
  Mux : Mux  Inputs=3
  Mux1 : Mux  Inputs=5
  Mux2 : Mux  Inputs=3
  SPI Master Transfer2 : raspberrypilib/SPI Master Transfer  Priority=6  BoardProperty=Pi 3 Model B  SPIModule=uint32(0)  Mode=Master  BusSpeed=1000000  Pin=SPI0_CE1  FirstBitToTransfer=Most significant bit (MSB)  ClockMode=0  BlockFunction=Transfer  RegisterAddress=0  OutputDataType=int8  OutputDataLength=1
      settings: SourceProductName=Simulink Support Package for Raspberry Pi Hardware  SourceProductBaseCode=RASPPI
  SPI_MSG_GET_ SENSOR offset : Constant  Value=12  OutMin=[1]  OutMax=[28]  OutDataTypeStr=uint8
  Sensor type offset : Constant  Value=8  OutDataTypeStr=uint8
  Sum : Sum  OutDataTypeStr=uint8
  Sum1 : Sum
  Valid data : Constant  Value=0  OutDataTypeStr=uint8
  Value : Outport
  Error : Outport  Port=2
  wires:
  SensorPort/1 -> Sum/1
  SensorType/1 -> Sum1/1
  0xA5/1 -> Equal2/1
  Sensor type offset/1 -> Sum1/2
  Sum1/1 -> Equal/1
  Equal2/1 -> Mux/1
  Mux/1 -> Error/1
  Equal/1 -> Mux/2
  Address3/1 -> Mux2/3
  Demux/3 -> Equal1/1
  Valid data/1 -> Equal1/2
  Demux/2 -> Equal/2
  Demux/1 -> Equal2/2
  Sum/1 -> Mux2/2
  SPI_MSG_GET_ SENSOR offset/1 -> Sum/2
  Mux2/1 -> SPI Master Transfer2/1
  Equal1/1 -> Mux/3
  SPI Master Transfer2/1 -> Bytes[3-6]/1
  "Address "/1 -> Mux2/1
  Bytes[3-6]/1 -> Demux/1
  Mux1/1 -> Value/1
  "Byte Packing "/1 -> Mux1/3, Mux1/2, Mux1/4, Mux1/5
  Constant/1 -> Mux1/1
  Demux/4 -> "Byte Packing "/2
  Demux/5 -> "Byte Packing "/1

== system BrickPi/Reset_all/Reset motor power/Reset power 1 ==
  note: Get sensor value
  note: Check whether 4th element == 0xA5?
  Power : Inport  OutDataTypeStr=int8
  0xA5 : Constant  Value=165
  "Address " : Constant  OutDataTypeStr=uint8
  Constant2 : Constant  OutDataTypeStr=uint8
  Constant3 : Constant  OutDataTypeStr=uint8
  Data Type Conversion : DataTypeConversion  OutDataTypeStr=uint8
  MotorPort1 : Constant  OutDataTypeStr=uint8
  Mux2 : Mux
  NAND : Logic  Operator=NAND  IconShape=distinctive  AllPortsSameDT=off  OutDataTypeStr=boolean
  SPI Master Transfer2 : raspberrypilib/SPI Master Transfer  Priority=6  BoardProperty=Pi 3 Model B  SPIModule=uint32(0)  Mode=Master  BusSpeed=1000000  Pin=SPI0_CE1  FirstBitToTransfer=Most significant bit (MSB)  ClockMode=0  BlockFunction=Transfer  RegisterAddress=0  OutputDataType=int8  OutputDataLength=1
      settings: SourceProductName=Simulink Support Package for Raspberry Pi Hardware  SourceProductBaseCode=RASPPI
  SPI_MSG_SET_ MOTOR_POWER : Constant  Value=21  OutMin=[1]  OutMax=[28]  OutDataTypeStr=uint8
  Selector1 : Selector  InputPortWidth=4  IndexOptions=Index vector (dialog)  Indices=[4]  OutputSizes=1
  Shift Arithmetic : ArithShift  BitShiftNumberSource=Input port  BitShiftNumber=8  BitShiftDirection=Left
      settings: InputPortMap=u0,p1
  Subtract : Sum  Inputs=+-
  Error : Outport
  wires:
  Subtract/1 -> Shift Arithmetic/2
  Mux2/1 -> SPI Master Transfer2/1
  "Address "/1 -> Mux2/1
  Constant3/1 -> Subtract/2
  MotorPort1/1 -> Subtract/1
  Constant2/1 -> Shift Arithmetic/1
  SPI_MSG_SET_ MOTOR_POWER/1 -> Mux2/2
  Data Type Conversion/1 -> Mux2/4
  Shift Arithmetic/1 -> Mux2/3
  Selector1/1 -> NAND/1
  NAND/1 -> Error/1
  SPI Master Transfer2/1 -> Selector1/1
  0xA5/1 -> NAND/2
  Power/1 -> Data Type Conversion/1

== system BrickPi/Reset_all/Reset motor power/Reset power 2 ==
  note: Get sensor value
  note: Check whether 4th element == 0xA5?
  Power : Inport  OutDataTypeStr=int8
  0xA5 : Constant  Value=165
  "Address " : Constant  OutDataTypeStr=uint8
  Constant2 : Constant  OutDataTypeStr=uint8
  Constant3 : Constant  OutDataTypeStr=uint8
  Data Type Conversion : DataTypeConversion  OutDataTypeStr=uint8
  MotorPort2 : Constant  Value=2  OutDataTypeStr=uint8
  Mux2 : Mux
  NAND : Logic  Operator=NAND  IconShape=distinctive  AllPortsSameDT=off  OutDataTypeStr=boolean
  SPI Master Transfer2 : raspberrypilib/SPI Master Transfer  Priority=6  BoardProperty=Pi 3 Model B  SPIModule=uint32(0)  Mode=Master  BusSpeed=1000000  Pin=SPI0_CE1  FirstBitToTransfer=Most significant bit (MSB)  ClockMode=0  BlockFunction=Transfer  RegisterAddress=0  OutputDataType=int8  OutputDataLength=1
      settings: SourceProductName=Simulink Support Package for Raspberry Pi Hardware  SourceProductBaseCode=RASPPI
  SPI_MSG_SET_ MOTOR_POWER : Constant  Value=21  OutMin=[1]  OutMax=[28]  OutDataTypeStr=uint8
  Selector1 : Selector  InputPortWidth=4  IndexOptions=Index vector (dialog)  Indices=[4]  OutputSizes=1
  Shift Arithmetic : ArithShift  BitShiftNumberSource=Input port  BitShiftNumber=8  BitShiftDirection=Left
      settings: InputPortMap=u0,p1
  Subtract : Sum  Inputs=+-
  Error : Outport
  wires:
  Subtract/1 -> Shift Arithmetic/2
  Mux2/1 -> SPI Master Transfer2/1
  "Address "/1 -> Mux2/1
  Constant3/1 -> Subtract/2
  MotorPort2/1 -> Subtract/1
  Constant2/1 -> Shift Arithmetic/1
  SPI_MSG_SET_ MOTOR_POWER/1 -> Mux2/2
  Data Type Conversion/1 -> Mux2/4
  Shift Arithmetic/1 -> Mux2/3
  Selector1/1 -> NAND/1
  NAND/1 -> Error/1
  SPI Master Transfer2/1 -> Selector1/1
  0xA5/1 -> NAND/2
  Power/1 -> Data Type Conversion/1

== system BrickPi/Reset_all/Reset motor power/Reset power 3 ==
  note: Get sensor value
  note: Check whether 4th element == 0xA5?
  Power : Inport  OutDataTypeStr=int8
  0xA5 : Constant  Value=165
  "Address " : Constant  OutDataTypeStr=uint8
  Constant2 : Constant  OutDataTypeStr=uint8
  Constant3 : Constant  OutDataTypeStr=uint8
  Data Type Conversion : DataTypeConversion  OutDataTypeStr=uint8
  MotorPort3 : Constant  Value=4  OutDataTypeStr=uint8
  Mux2 : Mux
  NAND : Logic  Operator=NAND  IconShape=distinctive  AllPortsSameDT=off  OutDataTypeStr=boolean
  SPI Master Transfer2 : raspberrypilib/SPI Master Transfer  Priority=6  BoardProperty=Pi 3 Model B  SPIModule=uint32(0)  Mode=Master  BusSpeed=1000000  Pin=SPI0_CE1  FirstBitToTransfer=Most significant bit (MSB)  ClockMode=0  BlockFunction=Transfer  RegisterAddress=0  OutputDataType=int8  OutputDataLength=1
      settings: SourceProductName=Simulink Support Package for Raspberry Pi Hardware  SourceProductBaseCode=RASPPI
  SPI_MSG_SET_ MOTOR_POWER : Constant  Value=21  OutMin=[1]  OutMax=[28]  OutDataTypeStr=uint8
  Selector1 : Selector  InputPortWidth=4  IndexOptions=Index vector (dialog)  Indices=[4]  OutputSizes=1
  Shift Arithmetic : ArithShift  BitShiftNumberSource=Input port  BitShiftNumber=8  BitShiftDirection=Left
      settings: InputPortMap=u0,p1
  Subtract : Sum  Inputs=+-
  Error : Outport
  wires:
  Subtract/1 -> Shift Arithmetic/2
  Mux2/1 -> SPI Master Transfer2/1
  "Address "/1 -> Mux2/1
  Constant3/1 -> Subtract/2
  MotorPort3/1 -> Subtract/1
  Constant2/1 -> Shift Arithmetic/1
  SPI_MSG_SET_ MOTOR_POWER/1 -> Mux2/2
  Data Type Conversion/1 -> Mux2/4
  Shift Arithmetic/1 -> Mux2/3
  Selector1/1 -> NAND/1
  NAND/1 -> Error/1
  SPI Master Transfer2/1 -> Selector1/1
  0xA5/1 -> NAND/2
  Power/1 -> Data Type Conversion/1

== system BrickPi/Reset_all/Reset motor power/Reset power 4 ==
  note: Get sensor value
  note: Check whether 4th element == 0xA5?
  Power : Inport  OutDataTypeStr=int8
  0xA5 : Constant  Value=165
  "Address " : Constant  OutDataTypeStr=uint8
  Constant2 : Constant  OutDataTypeStr=uint8
  Constant3 : Constant  OutDataTypeStr=uint8
  Data Type Conversion : DataTypeConversion  OutDataTypeStr=uint8
  MotorPort4 : Constant  Value=8  OutDataTypeStr=uint8
  Mux2 : Mux
  NAND : Logic  Operator=NAND  IconShape=distinctive  AllPortsSameDT=off  OutDataTypeStr=boolean
  SPI Master Transfer2 : raspberrypilib/SPI Master Transfer  Priority=6  BoardProperty=Pi 3 Model B  SPIModule=uint32(0)  Mode=Master  BusSpeed=1000000  Pin=SPI0_CE1  FirstBitToTransfer=Most significant bit (MSB)  ClockMode=0  BlockFunction=Transfer  RegisterAddress=0  OutputDataType=int8  OutputDataLength=1
      settings: SourceProductName=Simulink Support Package for Raspberry Pi Hardware  SourceProductBaseCode=RASPPI
  SPI_MSG_SET_ MOTOR_POWER : Constant  Value=21  OutMin=[1]  OutMax=[28]  OutDataTypeStr=uint8
  Selector1 : Selector  InputPortWidth=4  IndexOptions=Index vector (dialog)  Indices=[4]  OutputSizes=1
  Shift Arithmetic : ArithShift  BitShiftNumberSource=Input port  BitShiftNumber=8  BitShiftDirection=Left
      settings: InputPortMap=u0,p1
  Subtract : Sum  Inputs=+-
  Error : Outport
  wires:
  Subtract/1 -> Shift Arithmetic/2
  Mux2/1 -> SPI Master Transfer2/1
  "Address "/1 -> Mux2/1
  Constant3/1 -> Subtract/2
  MotorPort4/1 -> Subtract/1
  Constant2/1 -> Shift Arithmetic/1
  SPI_MSG_SET_ MOTOR_POWER/1 -> Mux2/2
  Data Type Conversion/1 -> Mux2/4
  Shift Arithmetic/1 -> Mux2/3
  Selector1/1 -> NAND/1
  NAND/1 -> Error/1
  SPI Master Transfer2/1 -> Selector1/1
  0xA5/1 -> NAND/2
  Power/1 -> Data Type Conversion/1

== system BrickPi/Reset_all/Reset sensor ports/Reset sensor port 1 ==
  note: Check whether 4th element == 0xA5?
  note: Set sensor type
  0xA5 : Constant  Value=165
  Address : Constant  VectorParams1D=off  OutDataTypeStr=uint8
  Mux1 : Mux
  NAND : Logic  Operator=NAND  IconShape=distinctive  AllPortsSameDT=off  OutDataTypeStr=boolean
  SPI Master Transfer1 : raspberrypilib/SPI Master Transfer  Priority=1  BoardProperty=Pi 3 Model B  SPIModule=uint32(0)  Mode=Master  BusSpeed=1000000  Pin=SPI0_CE1  FirstBitToTransfer=Most significant bit (MSB)  ClockMode=0  BlockFunction=Transfer  RegisterAddress=0  OutputDataType=int8  OutputDataLength=1
      settings: SourceProductName=Simulink Support Package for Raspberry Pi Hardware  SourceProductBaseCode=RASPPI
  SPI_MSG_SET_ SENSOR_TYPE : Constant  Value=12  OutMin=[1]  OutMax=[28]  OutDataTypeStr=uint8
  Selector1 : Selector  InputPortWidth=4  IndexOptions=Index vector (dialog)  Indices=[4]  OutputSizes=1
  SensorPort1 : Constant  OutDataTypeStr=uint8
  SensorTypeNone : Constant  OutDataTypeStr=uint8
  Error : Outport
  wires:
  Mux1/1 -> SPI Master Transfer1/1
  SPI Master Transfer1/1 -> Selector1/1
  Address/1 -> Mux1/1
  SPI_MSG_SET_ SENSOR_TYPE/1 -> Mux1/2
  SensorPort1/1 -> Mux1/3
  SensorTypeNone/1 -> Mux1/4
  Selector1/1 -> NAND/1
  0xA5/1 -> NAND/2
  NAND/1 -> Error/1

== system BrickPi/Reset_all/Reset sensor ports/Reset sensor port 2 ==
  note: Check whether 4th element == 0xA5?
  note: Set sensor type
  0xA5 : Constant  Value=165
  Address : Constant  VectorParams1D=off  OutDataTypeStr=uint8
  Mux1 : Mux
  NAND : Logic  Operator=NAND  IconShape=distinctive  AllPortsSameDT=off  OutDataTypeStr=boolean
  SPI Master Transfer1 : raspberrypilib/SPI Master Transfer  Priority=1  BoardProperty=Pi 3 Model B  SPIModule=uint32(0)  Mode=Master  BusSpeed=1000000  Pin=SPI0_CE1  FirstBitToTransfer=Most significant bit (MSB)  ClockMode=0  BlockFunction=Transfer  RegisterAddress=0  OutputDataType=int8  OutputDataLength=1
      settings: SourceProductName=Simulink Support Package for Raspberry Pi Hardware  SourceProductBaseCode=RASPPI
  SPI_MSG_SET_ SENSOR_TYPE : Constant  Value=12  OutMin=[1]  OutMax=[28]  OutDataTypeStr=uint8
  Selector1 : Selector  InputPortWidth=4  IndexOptions=Index vector (dialog)  Indices=[4]  OutputSizes=1
  SensorPort2 : Constant  Value=2  OutDataTypeStr=uint8
  SensorTypeNone : Constant  OutDataTypeStr=uint8
  Error : Outport
  wires:
  Mux1/1 -> SPI Master Transfer1/1
  SPI Master Transfer1/1 -> Selector1/1
  Address/1 -> Mux1/1
  SPI_MSG_SET_ SENSOR_TYPE/1 -> Mux1/2
  SensorPort2/1 -> Mux1/3
  SensorTypeNone/1 -> Mux1/4
  Selector1/1 -> NAND/1
  0xA5/1 -> NAND/2
  NAND/1 -> Error/1

== system BrickPi/Reset_all/Reset sensor ports/Reset sensor port 3 ==
  note: Check whether 4th element == 0xA5?
  note: Set sensor type
  0xA5 : Constant  Value=165
  Address : Constant  VectorParams1D=off  OutDataTypeStr=uint8
  Mux1 : Mux
  NAND : Logic  Operator=NAND  IconShape=distinctive  AllPortsSameDT=off  OutDataTypeStr=boolean
  SPI Master Transfer1 : raspberrypilib/SPI Master Transfer  Priority=1  BoardProperty=Pi 3 Model B  SPIModule=uint32(0)  Mode=Master  BusSpeed=1000000  Pin=SPI0_CE1  FirstBitToTransfer=Most significant bit (MSB)  ClockMode=0  BlockFunction=Transfer  RegisterAddress=0  OutputDataType=int8  OutputDataLength=1
      settings: SourceProductName=Simulink Support Package for Raspberry Pi Hardware  SourceProductBaseCode=RASPPI
  SPI_MSG_SET_ SENSOR_TYPE : Constant  Value=12  OutMin=[1]  OutMax=[28]  OutDataTypeStr=uint8
  Selector1 : Selector  InputPortWidth=4  IndexOptions=Index vector (dialog)  Indices=[4]  OutputSizes=1
  SensorPort3 : Constant  Value=4  OutDataTypeStr=uint8
  SensorTypeNone : Constant  OutDataTypeStr=uint8
  Error : Outport
  wires:
  Mux1/1 -> SPI Master Transfer1/1
  SPI Master Transfer1/1 -> Selector1/1
  Address/1 -> Mux1/1
  SPI_MSG_SET_ SENSOR_TYPE/1 -> Mux1/2
  SensorPort3/1 -> Mux1/3
  SensorTypeNone/1 -> Mux1/4
  Selector1/1 -> NAND/1
  0xA5/1 -> NAND/2
  NAND/1 -> Error/1

== system BrickPi/Reset_all/Reset sensor ports/Reset sensor port 4 ==
  note: Check whether 4th element == 0xA5?
  note: Set sensor type
  0xA5 : Constant  Value=165
  Address : Constant  VectorParams1D=off  OutDataTypeStr=uint8
  Mux1 : Mux
  NAND : Logic  Operator=NAND  IconShape=distinctive  AllPortsSameDT=off  OutDataTypeStr=boolean
  SPI Master Transfer1 : raspberrypilib/SPI Master Transfer  Priority=1  BoardProperty=Pi 3 Model B  SPIModule=uint32(0)  Mode=Master  BusSpeed=1000000  Pin=SPI0_CE1  FirstBitToTransfer=Most significant bit (MSB)  ClockMode=0  BlockFunction=Transfer  RegisterAddress=0  OutputDataType=int8  OutputDataLength=1
      settings: SourceProductName=Simulink Support Package for Raspberry Pi Hardware  SourceProductBaseCode=RASPPI
  SPI_MSG_SET_ SENSOR_TYPE : Constant  Value=12  OutMin=[1]  OutMax=[28]  OutDataTypeStr=uint8
  Selector1 : Selector  InputPortWidth=4  IndexOptions=Index vector (dialog)  Indices=[4]  OutputSizes=1
  SensorPort4 : Constant  Value=8  OutDataTypeStr=uint8
  SensorTypeNone : Constant  OutDataTypeStr=uint8
  Error : Outport
  wires:
  Mux1/1 -> SPI Master Transfer1/1
  SPI Master Transfer1/1 -> Selector1/1
  Address/1 -> Mux1/1
  SPI_MSG_SET_ SENSOR_TYPE/1 -> Mux1/2
  SensorPort4/1 -> Mux1/3
  SensorTypeNone/1 -> Mux1/4
  Selector1/1 -> NAND/1
  0xA5/1 -> NAND/2
  NAND/1 -> Error/1

== system BrickPi/Motor_Encoder/Get Encoder Value/Switch Case Action Subsystem/Subsystem ==
  MotorPort : Inport
  Enable : EnablePort
  Encoder : Subsystem
  Motor_Offset : Subsystem
  Terminator : Terminator
  wires:
  Encoder/1(Value) -> Motor_Offset/1(Offset)
  Encoder/2(Error) -> Terminator/1
  MotorPort/1 -> Motor_Offset/2(MotorPort), Encoder/1(MotorPort)

== system BrickPi/Motor_Status/Get motor values/Switch Case Action Subsystem/Subsystem ==
  MotorPort : Inport
  Enable : EnablePort
  Encoder : Subsystem
  Motor_Offset : Subsystem
  Terminator : Terminator
  wires:
  Encoder/1(Value) -> Motor_Offset/1(Offset)
  Encoder/2(Error) -> Terminator/1
  MotorPort/1 -> Motor_Offset/2(MotorPort), Encoder/1(MotorPort)

== system BrickPi/Motor_Encoder/Get Encoder Value/Switch Case Action Subsystem/Subsystem/Encoder ==
  note: Get motor encoder
  MotorPort : Inport
  0xA5 : Constant  Value=165
  "Address " : Constant  OutDataTypeStr=uint8
  Address3 : Constant  Value=[0 0 0 0 0 0 0 0]  OutDataTypeStr=uint8
  "Byte Packing " : xpcutilitieslib/Byte Packing   MaskPackedDataType=int32  MaskUnpackedDataTypes={'uint8', 'uint8', 'uint8', 'uint8'}  MaskAlignment=1
  Bytes[3-7] : Selector  IndexMode=Zero-based  InputPortWidth=10  IndexOptions=Index vector (dialog)  Indices=[3 4 5 6 7]  OutputSizes=1
  Demux : Demux  Outputs=5
  Mux2 : Mux  Inputs=3
  NAND : Logic  Operator=NAND  IconShape=distinctive  AllPortsSameDT=off  OutDataTypeStr=boolean
  SPI Master Transfer2 : raspberrypilib/SPI Master Transfer  Priority=6  BoardProperty=Pi 3 Model B  SPIModule=uint32(0)  Mode=Master  BusSpeed=1000000  Pin=SPI0_CE1  FirstBitToTransfer=Most significant bit (MSB)  ClockMode=0  BlockFunction=Transfer  RegisterAddress=0  OutputDataType=int8  OutputDataLength=1
      settings: SourceProductName=Simulink Support Package for Raspberry Pi Hardware  SourceProductBaseCode=RASPPI
  SPI_MSG_GET_ MOTOR_ENCODER offset : Constant  Value=29  OutDataTypeStr=uint8
  Sum : Sum  OutDataTypeStr=uint8
  Value : Outport
  Error : Outport  Port=2
  wires:
  Address3/1 -> Mux2/3
  NAND/1 -> Error/1
  Sum/1 -> Mux2/2
  Mux2/1 -> SPI Master Transfer2/1
  MotorPort/1 -> Sum/1
  Demux/5 -> "Byte Packing "/1
  "Address "/1 -> Mux2/1
  Demux/4 -> "Byte Packing "/2
  Demux/3 -> "Byte Packing "/3
  Demux/1 -> NAND/2
  0xA5/1 -> NAND/1
  Demux/2 -> "Byte Packing "/4
  "Byte Packing "/1 -> Value/1
  Bytes[3-7]/1 -> Demux/1
  SPI Master Transfer2/1 -> Bytes[3-7]/1
  SPI_MSG_GET_ MOTOR_ENCODER offset/1 -> Sum/2
